simulink model "Project_Lqr"  (R2021b)
settings: Solver=VariableStepAuto  StartTime=0.0  StopTime=500  RelTol=1e-3
undefined symbols (not defined in the file): A, B, C1, K
settings Model: Creator=nvnma  LastModifiedBy=nvnma

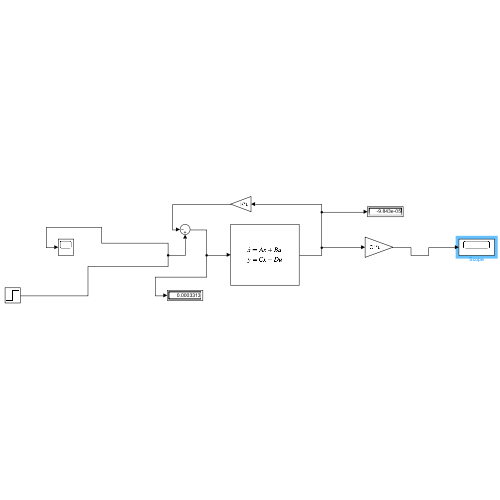
[thumbnail: Simulink's stored preview of the top-level diagram]
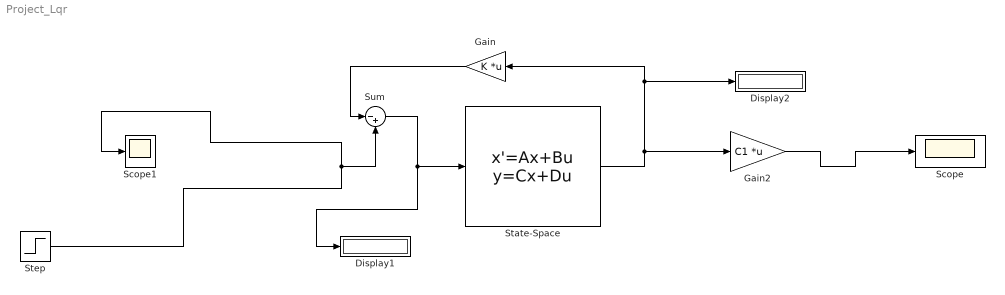
== system Project_Lqr ==
  Display1 : Display
  Display2 : Display
  Gain : Gain  Gain=K  Multiplication=Matrix(K*u)
  Gain2 : Gain  Gain=C1  Multiplication=Matrix(K*u)
  Scope : Scope
  Scope1 : Scope
  State-Space : StateSpace  A=A  B=B  C=eye(6)  D=[0 0 0 0 0 0]'  InitialCondition=[0 0 0 0 0 0]
  Step : Step  SampleTime=0
  Sum : Sum  Inputs=|-+
  wires:
  Sum/1 -> Display1/1, State-Space/1
  Step/1 -> Scope1/1, Sum/2
  Gain/1 -> Sum/1
  State-Space/1 -> Gain2/1, Display2/1, Gain/1
  Gain2/1 -> Scope/1
